simulink model "MPC4_QUES1"  (R2024b)
settings: Solver=VariableStepAuto  StartTime=0.0  StopTime=30  RelTol=1e-3
libraries: slpidlib x1
settings Model: Creator=Reza Shahriari  LastModifiedBy=Reza Shahriari
settings DebuggingCC: UnconnectedInputMsg=warning  UnconnectedOutputMsg=warning  UnconnectedLineMsg=warning
settings ModelReferenceCC: EnableRefExpFcnMdlSchedulingChecks=on
settings RTWCC: GPUComputeCapability=3.5  DLArmComputeVersion=19.05

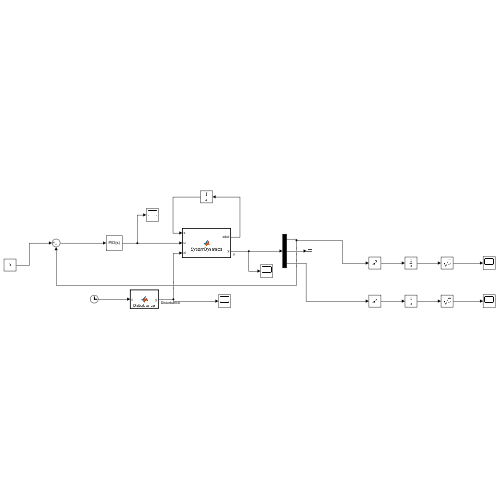
[thumbnail: Simulink's stored preview of the top-level diagram]
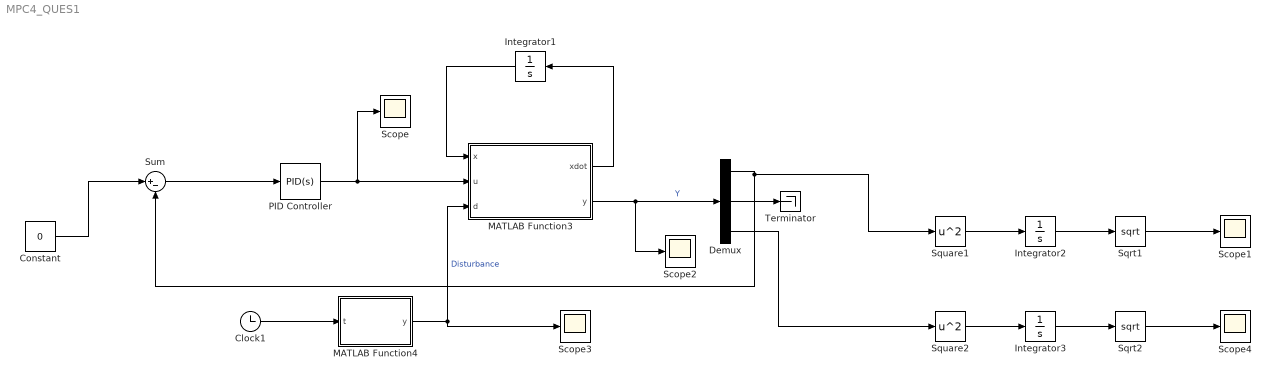
== system MPC4_QUES1 ==
  Clock1 : Clock
  Constant : Constant  Value=0
  Demux : Demux  Outputs=3
  Integrator1 : Integrator  InitialCondition=[0;0;0;0]
  Integrator2 : Integrator
  Integrator3 : Integrator
  MATLAB Function3 : MATLAB Function  TreatAsAtomicUnit=on
  MATLAB Function4 : MATLAB Function  TreatAsAtomicUnit=on
  PID Controller : slpidlib/PID Controller  Controller=PID  Form=Parallel  TimeDomain=Continuous-time  UseExternalTs=off  SampleTime=-1  IntegratorMethod=Forward Euler  FilterMethod=Forward Euler  ControllerParametersSource=internal  P=126134.015509655  I=126360.726224338  UseKiTs=off  D=30618.3678387567  UseExternalDerivativeSource=off  N=1487.32610581621  UseFilter=on  TunerSelectOption=Transfer Function Based (PID Tuner App)  InitialConditionSource=internal  InitialConditionForIntegrator=0  InitialConditionForFilter=0  DifferentiatorICPrevScaledInput=0  ExternalReset=none  TrackingMode=off  Kt=1  LimitOutput=off  SatLimitsSource=internal  UpperSaturationLimit=inf  LowerSaturationLimit=-inf  LinearizeAsGain=on  AntiWindupMode=none  Kb=1  LimitIntegrator=off  UpperIntegratorSaturationLimit=inf  LowerIntegratorSaturationLimit=-inf  POutMin=[]  POutMax=[]  IOutMin=[]  IOutMax=[]  DOutMin=[]  DOutMax=[]  NOutMin=[]  NOutMax=[]  SumOutMin=[]  SumOutMax=[]  SaturationOutMin=[]  SaturationOutMax=[]  PParamMin=[]  PParamMax=[]  IParamMin=[]  IParamMax=[]  DParamMin=[]  DParamMax=[]  NParamMin=[]  NParamMax=[]  KbParamMin=[]  KbParamMax=[]  KtParamMin=[]  KtParamMax=[]  KbOutMin=[]  KbOutMax=[]  KtOutMin=[]  KtOutMax=[]  IntegratorOutMin=[]  IntegratorOutMax=[]  FilterOutMin=[]  FilterOutMax=[]  SumI1OutMin=[]  SumI1OutMax=[]  SumI2OutMin=[]  SumI2OutMax=[]  SumI3OutMin=[]  SumI3OutMax=[]  SumI4OutMin=[]  SumI4OutMax=[]  SumDOutMin=[]  SumDOutMax=[]  DifferentiatorOutMin=[]  DifferentiatorOutMax=[]  FilterDiffOutCoefMin=[]  FilterDiffOutCoefMax=[]  ReciprocalOutMin=[]  ReciprocalOutMax=[]  SumDenOutMin=[]  SumDenOutMax=[]  SumNumOutMin=[]  SumNumOutMax=[]  DivideOutMin=[]  DivideOutMax=[]  UdiffTsProdOutMin=[]  UdiffTsProdOutMax=[]  NTsProdOutMin=[]  NTsProdOutMax=[]  UintegralTsProdOutMin=[]  UintegralTsProdOutMax=[]  UngainTsProdOutMin=[]  UngainTsProdOutMax=[]  ClampingZeroOutDataTypeStr=Inherit: Inherit via back propagation  ClampingZeroOutMin=[]  ClampingZeroOutMax=[]  FilterDenConstantOutDataTypeStr=Inherit: Inherit via back propagation  FilterDenConstantOutMin=[]  FilterDenConstantOutMax=[]  PCopyOutDataTypeStr=Inherit: Inherit via back propagation  PCopyOutMin=[]  PCopyOutMax=[]  NCopyOutDataTypeStr=Inherit: Inherit via back propagation  NCopyOutMin=[]  NCopyOutMax=[]  IntegratorContinuousStateAttributes=''  IntegratorStateMustResolveToSignalObject=off  IntegratorRTWStateStorageClass=Auto  FilterContinuousStateAttributes=''  FilterStateMustResolveToSignalObject=off  FilterRTWStateStorageClass=Auto  ParallelPVariant=InternalParameters  IdealPVariant=Disabled  IVariant=InternalParameters  DVariant=InternalParameters  IntegratorVariant=Continuous  SatVariant=Disabled  AWVariant=Passthrough  PCopyVariant=Disabled  TRVariant=Disabled  FdbkBlocksVariant=Forward  IdealPFdbkVariant=Disabled  SatFdbkVariant=Disabled  DerivativeFilterVariant=ContFilter  NVariant=InternalParameters  NCopyVariant=Disabled  FilterICVariant=InternalICsFilter  IntegratorICVariant=InternalICs  ExternalResetVariant=Disabled  TRSumVariant=Passthrough  SumFdbkVariant=Disabled  SumVariant=Sum_PID  TsampFilterVariant=InternalTs  TsampNgainVariant=Passthrough  TsampIntegralVariant=Disabled_SignalSpec  ExternalSaturationOutDataTypeStr=Inherit: Same as second input  DerivativeSourceVariant=ErrorSignal  PreIntVariant=InternalPreInt
  Scope{,1..4} (5 alike) : Scope
  Sqrt1 : Sqrt
  Sqrt2 : Sqrt
  Square1 : Math  Operator=square
  Square2 : Math  Operator=square
  Sum : Sum  Inputs=|+-
  Terminator : Terminator
  wires:
  MATLAB Function4/1(y) -> Scope3/1, MATLAB Function3/3(d)  "Disturbance"
  Clock1/1 -> MATLAB Function4/1(t)
  Integrator1/1 -> MATLAB Function3/1(x)
  MATLAB Function3/2(y) -> Demux/1, Scope2/1  "Y"
  MATLAB Function3/1(xdot) -> Integrator1/1
  Demux/2 -> Terminator/1
  Sum/1 -> PID Controller/1
  PID Controller/1 -> Scope/1, MATLAB Function3/2(u)
  Constant/1 -> Sum/1
  Sqrt1/1 -> Scope1/1
  Square1/1 -> Integrator2/1
  Integrator2/1 -> Sqrt1/1
  Demux/1 -> Square1/1, Sum/2
  Demux/3 -> Square2/1
  Square2/1 -> Integrator3/1
  Integrator3/1 -> Sqrt2/1
  Sqrt2/1 -> Scope4/1

== matlab function MPC4_QUES1/MATLAB Function3 ==
  data: x input; xdot output; u input; y output; d input
function [xdot,y]= SystemDynamics(x,u,d)

% Parameter Definition
Ms = 2500;
Mu = 320;
ks = 80000;
ku = 500000;
cs = 350;
cu = 15020;

A = [0 1 0 0;
     0 -cs/Ms -ks/Ms cs/Ms;
     0 1 0 -1;
     -ku/Mu cs/Mu (ks+ku)/Mu -(cs+cu)/Mu];
     
B = [0; 1/Ms; 0; -1/Mu];  % Input matrix

C = [1 0 0 0; 0 1 0 0; 0 0 1 0];

Ad = [0.9241    0.0945   -0.0672    0.0013;
   -2.0392    0.8450   -0.6570    0.0178;
    0.8830    0.0843   -0.1675    0.0021;
    1.2927    0.1390   -1.8258   -0.0591];

Bd = [    0.1053;
    2.2534;
   -0.8123;
  -51.0695];

Cd = C;


Diss = [0; cs*cu/(Ms*Mu); -cu/Mu; (cu/Mu)*(ku*cu-cs*Mu-cu*Mu)];

xdot = A*x + B*u + Diss*d;
y = C*x;

== matlab function MPC4_QUES1/MATLAB Function4 ==
  data: t input; y output
function y = Disturbance(t)

if t>=4 & t<5 
    y = t-4;
elseif t>=5 & t<7
    y = 1;
elseif t>=7 & t<8
    y = -t+8;
else 
    y = 0;
end
